simulink model "thrid_1_replacement1"  (R2021b)
settings: Solver=FixedStepAuto  StartTime=0.0  StopTime=10.0  RelTol=1e-3
settings Model: DataDictionary=thrid_1_replacement1_DD.sldd  DVDesignModelName=thrid_1  Creator=fredric  LastModifiedBy=fredric

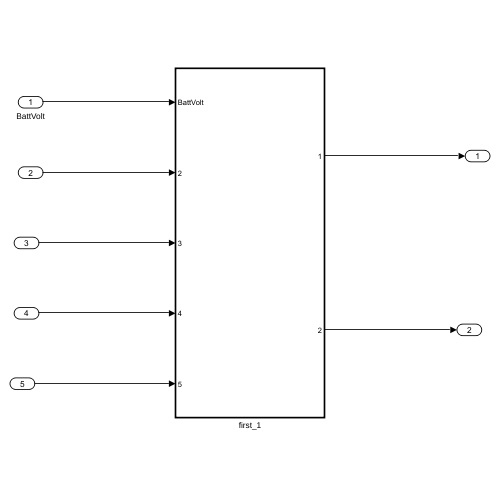
[thumbnail: Simulink's stored preview of the top-level diagram]
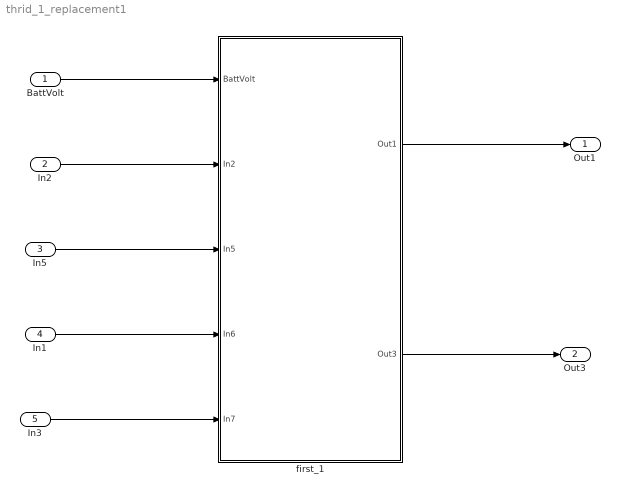
== system thrid_1_replacement1 ==
  BattVolt : Inport
  In2 : Inport  Port=2
  In5 : Inport  Port=3
  In1 : Inport  Port=4
  In3 : Inport  Port=5
  first_1 : Subsystem  TreatAsAtomicUnit=on  mask(Sldv ModelReference(Model name:first_1) Replacement){ModelName=first_1, ParameterArgumentNames=, ParameterArgumentValuesAsString=, SimulationMode=Accelerator}
      mask help: Replacement for the Model Reference block that references the model first_1. If Model arguments are specified on the Model Reference block, then they will appear in the mask parameters.
  Out1 : Outport
  Out3 : Outport  Port=2
  wires:
  BattVolt/1 -> first_1/1(BattVolt)
  In2/1 -> first_1/2(In2)
  In5/1 -> first_1/3(In5)
  In1/1 -> first_1/4(In6)
  In3/1 -> first_1/5(In7)
  first_1/1(Out1) -> Out1/1
  first_1/2(Out3) -> Out3/1

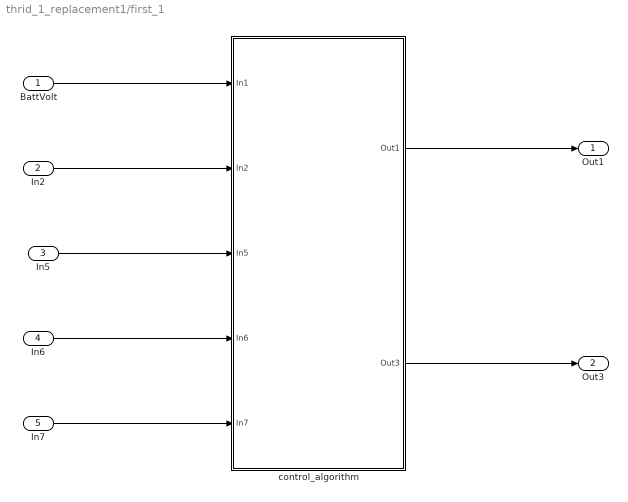
== system thrid_1_replacement1/first_1 ==
  BattVolt : Inport  OutDataTypeStr=double  PortDimensions=1
  In2 : Inport  Port=2  OutDataTypeStr=double  PortDimensions=1
  In5 : Inport  Port=3  OutDataTypeStr=double  PortDimensions=1
  In6 : Inport  Port=4  OutDataTypeStr=double  PortDimensions=1
  In7 : Inport  Port=5  OutDataTypeStr=double  PortDimensions=1
  control_algorithm : Subsystem
  Out1 : Outport  OutDataTypeStr=double  PortDimensions=1
  Out3 : Outport  Port=2  OutDataTypeStr=double  PortDimensions=1
  wires:
  control_algorithm/2(Out3) -> Out3/1
  control_algorithm/1(Out1) -> Out1/1
  In7/1 -> control_algorithm/5(In7)
  In6/1 -> control_algorithm/4(In6)
  In5/1 -> control_algorithm/3(In5)
  In2/1 -> control_algorithm/2(In2)
  BattVolt/1 -> control_algorithm/1(In1)

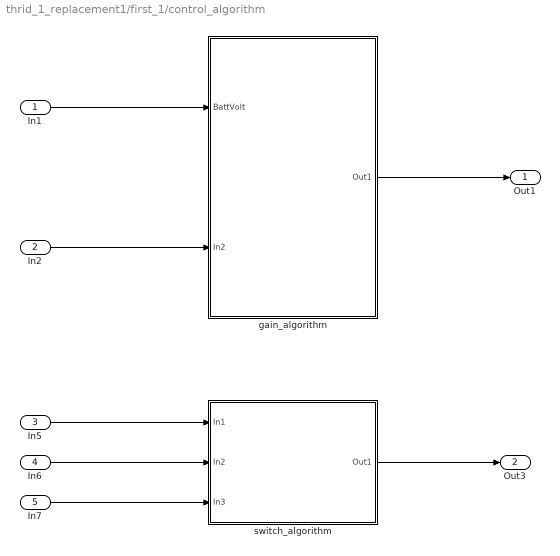
== system thrid_1_replacement1/first_1/control_algorithm ==
  In1 : Inport
  In2 : Inport  Port=2
  In5 : Inport  Port=3
  In6 : Inport  Port=4
  In7 : Inport  Port=5
  gain_algorithm : Subsystem
  switch_algorithm : Subsystem
  Out1 : Outport
  Out3 : Outport  Port=2
  wires:
  In1/1 -> gain_algorithm/1(BattVolt)
  In2/1 -> gain_algorithm/2(In2)
  gain_algorithm/1(Out1) -> Out1/1
  In5/1 -> switch_algorithm/1(In1)
  In6/1 -> switch_algorithm/2(In2)
  In7/1 -> switch_algorithm/3(In3)
  switch_algorithm/1(Out1) -> Out3/1

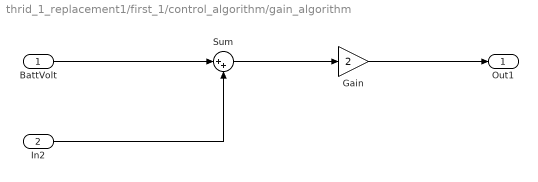
== system thrid_1_replacement1/first_1/control_algorithm/gain_algorithm ==
  BattVolt : Inport
  In2 : Inport  Port=2
  Gain : Gain  Gain=2
  Sum : Sum  Inputs=|++
  Out1 : Outport
  wires:
  Sum/1 -> Gain/1
  In2/1 -> Sum/2
  Gain/1 -> Out1/1
  BattVolt/1 -> Sum/1

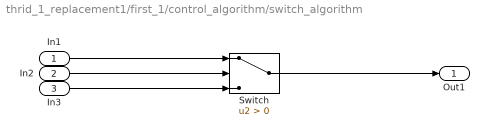
== system thrid_1_replacement1/first_1/control_algorithm/switch_algorithm ==
  In1 : Inport
  In2 : Inport  Port=2
  In3 : Inport  Port=3
  Switch : Switch  Criteria=u2 > Threshold
  Out1 : Outport
  wires:
  In3/1 -> Switch/3
  In2/1 -> Switch/2
  In1/1 -> Switch/1
  Switch/1 -> Out1/1
